simulink library "carnot"  (R2018b)
settings: Solver=VariableStepAuto  StartTime=0.0  StopTime=10.0  RelTol=1e-3
undefined symbols (not defined in the file or in its folder): A, A_earth, acol, Acol, ActPower1, ActPower2, ActPower3, Ad, Ad0, Ar, Au, Au0, Azimuth_Angle, B, Bd, Bd0, Br, Bu, Bu0, C, c1, c2, c3, c33, c4, c5, c6, CarnotCallbacks_Density, CarnotCallbacks_Enthalpy, CarnotCallbacks_Enthalpy2Temperature, CarnotCallbacks_Entropy, CarnotCallbacks_Evaporation_Enthalpy, CarnotCallbacks_GlobalMessageLevel, CarnotCallbacks_Grashof, CarnotCallbacks_Heat_Capacity, CarnotCallbacks_Kinematic_Viscosity, CarnotCallbacks_PMV_PPD, CarnotCallbacks_Prandtl, CarnotCallbacks_Saturation_Property, CarnotCallbacks_Saturation_Temperature, CarnotCallbacks_Saturation_Value_Water, CarnotCallbacks_Specific_Volume, CarnotCallbacks_Thermal_Conductivity, CarnotCallbacks_Vapour_Content, CarnotCallbacks_Vapour_Pressure, Cd, Cdl, Cr, Cu, Davies, Dd, DE_TRY2010_04_averageYear, delta_grd, density, DiameterLastPiece, dl, DPConstant, DPLinear, DPQuadratic, Dr ... (+59)
libraries: $bdroot x429, simulink x36, simulink_extras x12
(part 19 of 22)

== system carnot/Storage/Thermal/Storage_Type_5 ==
  note: Domestic hot water heat exchanger
  note: pipe connection to charge DHW section
  note: pipe connection for house heating
  note: pipe connection to charge house heating section
  note: heat exchanger solar
  note: heat exchanger for DHW circulation
  Tamb : Inport
  THB_dhw : Inport  Port=2
  THB_chg_up : Inport  Port=3
  THB_dis_mid : Inport  Port=4
  THB_chg_mid : Inport  Port=5
  THB_hx_low : Inport  Port=6
  THB_circ : Inport  Port=7
  Pel : Inport  Port=8
  Constant_THB : $bdroot/Source/Simple/Constant_THB  t=20  mdot=0  p=1e5  mID=No Pressure Drop  fluid=Water  mix=0  mix2=0  mix3=0  dia=0.02  hgt=0
  CreateSdat : $bdroot/Basic/Thermal_Models/CreateSdat  volume=volume  stgtype=stgtype
  Electric_Heating_1 : $bdroot/Storage/Thermal/Storage_Ports/Electric_Heating  hin=heater1start  hout=heater1end  nodes=nodes
  HX_EN12977_1 : $bdroot/Storage/Thermal/Storage_Ports/HX_EN12977  h_in=hx1inlet  h_out=hx1outlet  hgt=hgt  dia=hx1dia  height=-0.70492  ua0=hx1uac  uam=hx1uam  uat=hx1uat  uat2=hx1_uat2  dplin=hx1dplin  dpqua=hx1dpqua  nodes=nodes
  HX_EN12977_2 : $bdroot/Storage/Thermal/Storage_Ports/HX_EN12977  h_in=hx2inlet  h_out=hx2outlet  hgt=hgt  dia=hx2dia  height=1.7623  ua0=hx2uac  uam=hx2uam  uat=hx2uat  uat2=hx2_uat2  dplin=hx2dplin  dpqua=hx2dpqua  nodes=nodes
  HX_EN12977_3 : Subsystem  mask(heat exchanger for storage, data EN 12977){h_in=hx3inlet, h_out=hx3outlet, hgt=hgt, dia=hx3dia, height=0.17623, ua0=hx3uac, uam=hx3uam, uat=hx3uat, uat2=hx3_uat2, dplin=hx3dplin, dpqua=hx3dpqua, nodes=nodes}
      mask prompts: h_in "relative height of inlet"; h_out "relative height of outlet"; hgt "Height of storage in m"; dia "Diameter of HX pipe [m]"; height "Height difference inlet-outlet [m]"; ua0 "uac: heat transfer coefficient [W/K /(kg/s) /(°C)]"; uam "uam: massflow dependent heat transfer [-]"; uat "uat: temperature dependent heat transfer [-]"; uat2 "uat2: temperature difference dependent heat transfer [-]"; dplin "Pressure drop coefficient dplin [Pa/(kg/s)]"; dpqua "Pressure drop coefficient dpqua [Pa/(kg/s)²]"; nodes "number of nodes"
      mask help:
      | The block transforms the incoming THV vector to a vector which the storage interprets as a heat exchanger.
      | Give inlet and outlet as a relative position 0=bottom to 1=top
      | The heat transfer is calculated by:
      | UA = uac * mdot^uam *
      |           ((Theatexchanger+Tstorage)/2)^uat *
      |           (Theatexchanger-Tstorage)^uat2
      mask init: same as carnot/Storage/Thermal/Storage_Ports/HX_EN12977
      mask Help: web(['file:///' fullfile(path_carnot('help'),'StoragePorts_HeatExchangerModels.html')],'-helpbrowser')
      mask TypeOptions dia: Pressure_Drop_StorageHX/dia
      mask TypeOptions height: Pressure_Drop_StorageHX/hgt
      mask TypeOptions ua0: sfun_storage_heatexchanger/p1
      mask TypeOptions uam: sfun_storage_heatexchanger/p2
      mask TypeOptions uat: sfun_storage_heatexchanger/p3
      mask TypeOptions uat2: sfun_storage_heatexchanger/p4
      mask TypeOptions dplin: Pressure_Drop_StorageHX/dplin
      mask TypeOptions dpqua: Pressure_Drop_StorageHX/dpqua
      mask TypeOptions nodes: sfun_storage_heatexchanger/nodes
      mask DialogControl ParameterTabVar0 Prompt: Geometry
      mask DialogControl ParameterTabVar01 Prompt: Heat transfer
      mask DialogControl ParameterTabVar012 Prompt: Pressure drop
      mask DialogControl ParameterTabVar0123 Prompt: Calculation
      mask Display: disp('HX EN12977')
  Pipe_Connection_1 : $bdroot/Storage/Thermal/Storage_Ports/Pipe_Connection  h_in=pipe1inlet  h_out=pipe1outlet  hgt=hgt  dpipe=pipe1dia  dstg=dia  height=-0.17623  nodes=nodes
  Pipe_Connection_2 : $bdroot/Storage/Thermal/Storage_Ports/Pipe_Connection  h_in=pipe2inlet  h_out=pipe2outlet  hgt=hgt  dpipe=pipe2dia  dstg=dia  height=0.17623  nodes=nodes
  Pipe_Connection_3 : $bdroot/Storage/Thermal/Storage_Ports/Pipe_Connection  h_in=pipe3inlet  h_out=pipe3outlet  hgt=hgt  dpipe=pipe3dia  dstg=dia  height=-0.70492  nodes=nodes
  T_Sensor_Surface : $bdroot/Control/T_Sensor_Surface  pos=Tsensor  tdel=10  t0=mean(tini)
  select_T : Selector  InputPortWidth=nodes  IndexOptions=Index vector (dialog)  Indices=[1 3 5 7 9 11 13 15 17 19]  OutputSizes=1
  sfun_storageTnodes : $bdroot/Basic/Thermal_Models/sfun_storageTnodes  uloss=uwall  ubot=ubot  utop=utop  cond=axcond  volume=volume  dia=dia  standing=standing cylinder  tini=tini  nodes=nodes  nconnect=7  elimthermocline=2  condinvtc=1e5
  Sdat : Outport
  Tsensors : Outport  Port=2
  THBdhw : Outport  Port=3
  THBchg_up : Outport  Port=4
  THBdis_mid : Outport  Port=5
  THBchg_mid : Outport  Port=6
  THBhx_low : Outport  Port=7
  THBcirc : Outport  Port=8
  wires:
  Electric_Heating_1/1 -> sfun_storageTnodes/8
  Pel/1 -> CreateSdat/20, Electric_Heating_1/1
  HX_EN12977_3/2(THBout) -> CreateSdat/19, THBcirc/1  "THBoutHX3"
  HX_EN12977_3/1(to_storeT) -> sfun_storageTnodes/7
  THB_circ/1 -> CreateSdat/18, HX_EN12977_3/2(THBin)  "THBinHX3"
  T_Sensor_Surface/1 -> Tsensors/1
  HX_EN12977_1/2 -> CreateSdat/15, THBhx_low/1  "THBoutHX1"
  THB_hx_low/1 -> CreateSdat/14, HX_EN12977_1/2  "THBinHX1"
  Pipe_Connection_3/1 -> sfun_storageTnodes/3
  Pipe_Connection_3/2 -> THBchg_up/1, CreateSdat/9  "THBoutPipe3"
  THB_chg_up/1 -> CreateSdat/8, Pipe_Connection_3/2  "THBinPipe3"
  CreateSdat/1 -> Sdat/1
  sfun_storageTnodes/2 -> T_Sensor_Surface/1, select_T/1, HX_EN12977_2/1, Pipe_Connection_3/1, Pipe_Connection_1/1, HX_EN12977_3/1(from_storeT), HX_EN12977_1/1, Pipe_Connection_2/1  "Tnodes"
  select_T/1 -> CreateSdat/3  "Tnodes"
  HX_EN12977_2/1 -> sfun_storageTnodes/2
  HX_EN12977_2/2 -> CreateSdat/17, THBdhw/1  "THBoutHX2"
  THB_dhw/1 -> CreateSdat/16, HX_EN12977_2/2  "THBinHX2"
  Tamb/1 -> sfun_storageTnodes/1, CreateSdat/1  "Tamb"
  THB_dis_mid/1 -> Pipe_Connection_2/2, CreateSdat/6  "THBinPipe2"
  Pipe_Connection_2/1 -> sfun_storageTnodes/4
  Pipe_Connection_2/2 -> THBdis_mid/1, CreateSdat/7  "THBoutPipe2"
  HX_EN12977_1/1 -> sfun_storageTnodes/6
  THB_chg_mid/1 -> CreateSdat/4, Pipe_Connection_1/2, Electric_Heating_1/2  "THBinPipe1"
  Pipe_Connection_1/1 -> sfun_storageTnodes/5
  Pipe_Connection_1/2 -> THBchg_mid/1, CreateSdat/5  "THBoutPipe1"
  sfun_storageTnodes/1 -> CreateSdat/2  "Energy"
  Constant_THB/1 -> CreateSdat/10, CreateSdat/12, CreateSdat/13, CreateSdat/11

== system carnot/Storage/Thermal/detailed_storage_models ==
  heat_exchanger_storage : Subsystem  mask(storage with heat exchanger){v=[0.002 0.0005], loss=0.1, uh=[500 1], uc=[500 1], uw=[300 1], mat=aluminium, m=[3 0.1], t0=20, dph=[200 100 1], dpc=[20 10 0.5], n=1}
      mask prompts: v "volume [exchanger storage] [m³]"; loss "ua losses [W/K]"; uh "heat transfer in exchanger [constant linear_in_massflow] [W/K]"; uc "heat transfer to storage [constant linear_massflow] [W/K]"; uw "heat transfer to wall [constant linear_in_massflow] [W/K]"; mat "material"; m "[mass_in_kg fraction_exchanger]"; t0 "initial temperature [degree centigrade]"; dph "pressure drop exchanger [linear quadratic lin_T] [Pa]"; dpc "pressure drop storage [linear quadratic lin_T] [Pa]"; n "number of nodes"
      mask help: This block is a heat exchanger, taking the fluid volume of the cold and hot side and the thermal capacity of the walls into account.
      mask init:
      | v = max(0.00001, v);
      | n = max(n,1);
      mask Help: web(fullfile(path_carnot('help'),'heat_exchanger_storage.html'),'-helpbrowser')
      mask TypeOptions mat: aluminium | bronze | cast iron | steel | stainless steel | copper | brass | gravel | granite | glass | PU-foam | glass wool
      mask Display: plot(0,-10,110,95,[30,30,35,65,70,70,65,35,30],[90,60,54,54,60,90,95,95,90],[30,66,34,66,34,66,30],[63,63,68,73,76,81,81])

== system carnot/Storage/Thermal/surface_models ==
  Isolated_Cover : Subsystem  mask(isolated cover){u=0.6}
      mask prompts: u "loss coefficient of isolation [W/(m²*K)]"
      mask help: This is a surface-model for ground storages. It describes the absorption of solar radiation and the heat losses by wind.
      mask Help: web(fullfile(path_carnot('help'),'Isolated_Cover.html'),'-helpbrowser')
  Open_Surface : Subsystem  mask(open surface){albedo=0.6}
      mask prompts: albedo "albedo of the surface [0..1]"
      mask help: This is a surface-model for ground storages. It describes the absorption of solar radiation and the heat losses by wind.
      mask init:
      | albedo = min(1, max(0, albedo));
      mask Help: web(fullfile(path_carnot('help'),'Open_Surface.html'),'-helpbrowser')

== system carnot/Basic/Heat_Transfer/alfa_window_in/Shading ==
  WDB : Inport
  control : Inport  Port=2
  Bus Selector : BusSelector  OutputSignals=Zenith_Angle
  Demux : Demux
  Mux : Mux  Inputs=2
  S-Function : S-Function  FunctionName=venetian  Parameters=bli_a, bli_b, bli_c, bli_d, bli_alpha, bli_refl, shad_type, type_glazing, tau_shad  SFunctionDeploymentMode=off  EnableBusSupport=off
  f_dir : Outport
  f_dfu : Outport  Port=2
  f_g : Outport  Port=3
  f_tau : Outport  Port=4
  wires:
  WDB/1 -> Bus Selector/1
  Bus Selector/1 -> Mux/2  "<Zenith_Angle>"
  control/1 -> Mux/1
  Mux/1 -> S-Function/1
  S-Function/1 -> Demux/1
  Demux/1 -> f_dir/1
  Demux/2 -> f_dfu/1
  Demux/3 -> f_g/1
  Demux/4 -> f_tau/1

== system carnot/Basic/Heat_Transfer/alfa_window_in/Subsystem ==
  note: 1. solar radiation into room (behind window glass layers)
      | 2. absorbed solar radiation flowing from inner window surface into zone
  note: TAUALFA 1-2-3-4 layers,standardized to 1.0,(4 mm float glass, no dirt absorption,97% room absorption)
      | The TAUALFA-Lookup-table is calculated with "taualfa.m"
  note: Assumption:
      | 1. gvalue = gvalue(0)
      | 2. gvalue(teta) / gvalue = tau(teta) / tau(0)
  sun_t : Inport
  In2 : Inport  Port=2
  In3 : Inport  Port=3
  In4 : Inport  Port=4
  In5 : Inport  Port=5
  2-D Lookup Table : Lookup_n-D  BreakpointsForDimension1=[0:10:90]  BreakpointsForDimension2=[1:4]  Table=[1.0000 1.0000 1.0000 1.0000; 0.9996 0.9991 0.9987 0.9983; 0.9979 0.9961 0.9945 0.9929; 0.9937 0.9894 0.9861 0.9836; 0.9839 0.9753 0.9704 0.9680; 0.9608 0.9438 0.9365 0.9361; 0.9061 0.8679 0.8484 0.8413; 0.7755 0.6821 0.6182 0.5717; 0.4807 0.3277 0.2324 0.1688; 0 0 0 0]  InternalRulePriority=Speed  RndMeth=Simplest  InputSameDT=on
  Demux2 : Demux  Outputs=2
  Demux3 : Demux  Outputs=3
  Mux2 : Mux  Inputs=2
  Product{1..3,7..8} (5 alike) : Product  SaturateOnIntegerOverflow=on  RndMeth=Zero  InputSameDT=on  OutDataTypeStr=Inherit: Same as first input
  Product11 : Product  Inputs=3  SaturateOnIntegerOverflow=on  RndMeth=Zero  InputSameDT=on  OutDataTypeStr=Inherit: Same as first input
  Sum4 : Sum  Inputs=+-  SaturateOnIntegerOverflow=on  InputSameDT=on  OutDataTypeStr=Inherit: Same as first input
  Sum5 : Sum  SaturateOnIntegerOverflow=on  InputSameDT=on  OutDataTypeStr=Inherit: Same as first input
  const1 : Constant  Value=gvalue
  numlayer : Constant  Value=numlayer
  tau(0) : Gain  Gain=tauzero  SaturateOnIntegerOverflow=on  OutDataTypeStr=Inherit: Same as input  ParamDataTypeStr=Inherit: Same as input
  tau,dfu - angle : Constant  Value=60
  qdot_abs : Outport
  qdot_sol : Outport  Port=2
  wires:
  In5/1 -> Product3/2
  In2/1 -> Product2/2
  Sum4/1 -> qdot_abs/1
  Demux2/2 -> Product8/1  "tau_norm(60)"
  numlayer/1 -> 2-D Lookup Table/2
  Demux2/1 -> Product7/1  "tau_norm(teta)"
  In4/1 -> Product11/3
  Product11/1 -> Sum4/1  "qdot_room"
  Product7/1 -> Sum5/1
  Sum5/1 -> Product11/2, tau(0)/1
  Product3/1 -> Sum4/2, qdot_sol/1
  Product8/1 -> Sum5/2
  Product2/1 -> Product7/2
  tau(0)/1 -> Product3/1
  tau,dfu - angle/1 -> Mux2/2
  Demux3/3 -> Product1/1  "Idfu_t"
  const1/1 -> Product11/1
  Demux3/2 -> Product2/1  "Idir_t"
  Demux3/1 -> Mux2/1  "teta"
  Mux2/1 -> 2-D Lookup Table/1
  In3/1 -> Product1/2
  sun_t/1 -> Demux3/1
  2-D Lookup Table/1 -> Demux2/1
  Product1/1 -> Product8/2

== system carnot/Basic/Hydraulics/Flow_Mixer_basic/Subsystem ==
  clq_bus : Inport
  Bus Selector10 : BusSelector  OutputSignals=MassFlow,DPConstant,DPLinear,DPQuadratic
  Mux : Mux
  clq : Outport
  wires:
  Mux/1 -> clq/1
  clq_bus/1 -> Bus Selector10/1
  Bus Selector10/4 -> Mux/4  "<DPQuadratic>"
  Bus Selector10/3 -> Mux/3  "<DPLinear>"
  Bus Selector10/2 -> Mux/2  "<DPConstant>"
  Bus Selector10/1 -> Mux/1  "<MassFlow>"

== system carnot/Basic/Hydraulics/Flow_Mixer_basic/Subsystem1 ==
  THB : Inport
  Bus Selector1 : BusSelector  OutputSignals=ID,DPConstant,DPLinear,DPQuadratic
  Mux : Mux
  IDclq : Outport
  wires:
  Bus Selector1/4 -> Mux/4  "<DPQuadratic>"
  Bus Selector1/3 -> Mux/3  "<DPLinear>"
  Bus Selector1/2 -> Mux/2  "<DPConstant>"
  Bus Selector1/1 -> Mux/1  "<ID>"
  Mux/1 -> IDclq/1
  THB/1 -> Bus Selector1/1

== system carnot/Basic/Hydraulics/Flow_Mixer_basic/Subsystem2 ==
  THB : Inport
  Bus Selector1 : BusSelector  OutputSignals=ID,DPConstant,DPLinear,DPQuadratic
  Mux : Mux
  IDclq : Outport
  wires:
  THB/1 -> Bus Selector1/1
  Mux/1 -> IDclq/1
  Bus Selector1/1 -> Mux/1  "<ID>"
  Bus Selector1/2 -> Mux/2  "<DPConstant>"
  Bus Selector1/3 -> Mux/3  "<DPLinear>"
  Bus Selector1/4 -> Mux/4  "<DPQuadratic>"

== system carnot/Basic/Hydraulics/Flow_Mixer_basic/average_1 ==
  In1 : Inport
  In2 : Inport  Port=2
  average2 : Gain  Gain=0.5  SaturateOnIntegerOverflow=on  OutDataTypeStr=Inherit: Same as input  ParamDataTypeStr=Inherit: Same as input
  sum2 : Sum  SaturateOnIntegerOverflow=on  InputSameDT=on  OutDataTypeStr=Inherit: Same as first input
  Out1 : Outport
  wires:
  In1/1 -> sum2/1
  average2/1 -> Out1/1
  sum2/1 -> average2/1
  In2/1 -> sum2/2

== system carnot/Basic/Hydraulics/Flow_Mixer_basic/decrease_ID1 ==
  In1 : Inport
  Abs : Abs
  Bias : Bias  Bias=-1
  Dot Product1 : DotProduct  InputSameDT=on  OutDataTypeStr=Inherit: Inherit via internal rule
  Sign : Signum
  Out1 : Outport
  wires:
  Bias/1 -> Dot Product1/2
  Sign/1 -> Dot Product1/1
  Abs/1 -> Bias/1
  Dot Product1/1 -> Out1/1
  In1/1 -> Sign/1, Abs/1

== system carnot/Basic/Hydraulics/Flow_Mixer_basic/decrease_ID2 ==
  In1 : Inport
  Abs : Abs
  Bias : Bias  Bias=-1
  Dot Product1 : DotProduct  InputSameDT=on  OutDataTypeStr=Inherit: Inherit via internal rule
  Sign : Signum
  Out1 : Outport
  wires:
  In1/1 -> Abs/1, Sign/1
  Dot Product1/1 -> Out1/1
  Abs/1 -> Bias/1
  Sign/1 -> Dot Product1/1
  Bias/1 -> Dot Product1/2

== system carnot/Basic/Hydraulics/Mix_T_Mdot/select1 ==
  In1 : Inport
  Bus Selector1 : BusSelector  OutputSignals=Temperature,MassFlow,Pressure,FluidType,FluidMix
  Mux : Mux  Inputs=5
  Out1 : Outport
  wires:
  Mux/1 -> Out1/1
  In1/1 -> Bus Selector1/1
  Bus Selector1/5 -> Mux/5  "<FluidMix>"
  Bus Selector1/4 -> Mux/4  "<FluidType>"
  Bus Selector1/3 -> Mux/3  "<Pressure>"
  Bus Selector1/2 -> Mux/2  "<MassFlow>"
  Bus Selector1/1 -> Mux/1  "<Temperature>"

== system carnot/Basic/Hydraulics/Mix_T_Mdot/select2 ==
  In1 : Inport
  Bus Selector1 : BusSelector  OutputSignals=Temperature,MassFlow,Pressure,FluidType,FluidMix
  Mux : Mux  Inputs=5
  Out1 : Outport
  wires:
  Bus Selector1/1 -> Mux/1  "<Temperature>"
  Bus Selector1/2 -> Mux/2  "<MassFlow>"
  Bus Selector1/3 -> Mux/3  "<Pressure>"
  Bus Selector1/4 -> Mux/4  "<FluidType>"
  Bus Selector1/5 -> Mux/5  "<FluidMix>"
  In1/1 -> Bus Selector1/1
  Mux/1 -> Out1/1

== system carnot/Basic/Pressure_Drop/Pressure_Drop/calculate_dp ==
  THBin : Inport
  c : Inport  Port=2
  l : Inport  Port=3
  q : Inport  Port=4
  Enable : EnablePort
  Bus Selector : BusSelector  OutputSignals=DPConstant
  Bus Selector2 : BusSelector  OutputSignals=DPLinear
  Bus Selector3 : BusSelector  OutputSignals=DPQuadratic
  Bus Selector5 : BusSelector  OutputSignals=MassFlow
  Math Function : Math  Operator=square  SaturateOnIntegerOverflow=on
  Product : Product
  Product1 : Product
  sum : Sum  SaturateOnIntegerOverflow=on  InputSameDT=on  OutDataTypeStr=Inherit: Same as first input
  sum2 : Sum  SaturateOnIntegerOverflow=on  InputSameDT=on  OutDataTypeStr=Inherit: Same as first input
  sum3 : Sum  SaturateOnIntegerOverflow=on  InputSameDT=on  OutDataTypeStr=Inherit: Same as first input
  sum4 : Sum  Inputs=3  SaturateOnIntegerOverflow=on  InputSameDT=on  OutDataTypeStr=Inherit: Same as first input
  dp : Outport
  con : Outport  Port=2
  lin : Outport  Port=3
  qua : Outport  Port=4
  wires:
  sum3/1 -> qua/1
  sum2/1 -> lin/1
  sum/1 -> con/1
  Product/1 -> sum4/2
  Product1/1 -> sum4/1
  Bus Selector2/1 -> sum2/2  "<DPLinear>"
  Bus Selector/1 -> sum/2  "<DPConstant>"
  Bus Selector3/1 -> sum3/2  "<DPQuadratic>"
  Math Function/1 -> Product1/1
  sum4/1 -> dp/1
  Bus Selector5/1 -> Product/1, Math Function/1  "<MassFlow>"
  THBin/1 -> Bus Selector/1, Bus Selector2/1, Bus Selector3/1, Bus Selector5/1
  l/1 -> Product/2, sum2/1
  c/1 -> sum4/3, sum/1
  q/1 -> Product1/2, sum3/1

== system carnot/Basic/Pressure_Drop/Pressure_Drop_PipeTheory/DP_Geometry ==
  Tnodes : Inport
  mdot : Inport  Port=2
  Enable : EnablePort
  Bus Selector4 : BusSelector  OutputSignals=MassFlow,Pressure,FluidType,FluidMix
  S-Function : S-Function  FunctionName=pipe_PressureDrop  Parameters="dia, len,  rough, nbend"  SFunctionDeploymentMode=off  EnableBusSupport=off
  lin : Outport  OutputWhenDisabled=reset  InitialOutput=0
  qua : Outport  Port=2  OutputWhenDisabled=reset  InitialOutput=0
  dp : Outport  Port=3  OutputWhenDisabled=reset  InitialOutput=0
  wires:
  Tnodes/1 -> S-Function/1
  S-Function/1 -> lin/1
  S-Function/2 -> qua/1
  mdot/1 -> Bus Selector4/1
  Bus Selector4/1 -> S-Function/2  "<MassFlow>"
  Bus Selector4/2 -> S-Function/3  "<Pressure>"
  Bus Selector4/3 -> S-Function/4  "<FluidType>"
  Bus Selector4/4 -> S-Function/5  "<FluidMix>"
  S-Function/3 -> dp/1

== system carnot/Basic/Pressure_Drop/Pressure_Drop_changeD/2//pi//d^2//density ==
  note: sudden increase in diameter (A1 < A2)
      |   for a flow from A1 to A2
      |   zeta = (1 - A1/A2)^2 = (1 - (d1/d2)^2)^2
      | sudden decrease in diameter (A1 < A2)
      |   for a flow from A2 to A1
      |   zeta = 0.5 * (1 - A1/A2)^2 = 0.5 * (1 - (d1/d2)^2)^2
      | dp = zeta * density/2 * w^2
      | dp = c + l*mdot + q*mdot^2    Carnot approach (here c = l = 0)
      | with mdot = Vdot*density = w*A*density  -> w = mdot/A/density
      | dp = zeta * density/2 * mdot^2/A^2/density^2
      | dp = zeta/(2*A^2*density) * mdot^2
      | -> q = zeta/(2*A^2*density)
      | diameter increase:
      |   q = (1 - A1/A2)^2/(2*A1^2*density)
      |   q = (1/A1 - 1/A2)^2 / (2*density)
      |   with A = pi/4*d^2
      |   q = 8/density/pi^2 * (1/d1^2 - 1/d2^2)^2
      | diameter decrease:
      |   q = 0.5*(1 - A1/A2)^2/(2*A1^2*density)
      |   q = 0.5*(1/A1 - 1/A2)^2 / (2*density)
      |   with A = pi/4*d^2
      |   q = 4/density/pi^2 * (1/d1^2 - 1/d2^2)^2
  THB : Inport
  Enable : EnablePort
  Abs : Abs
  Add : Sum  Inputs=+-
  Bus Selector3 : BusSelector  OutputSignals=DiameterLastPiece
  Constant : Constant  Value=dia
  Constant1 : Constant  Value=8
  Constant2 : Constant  Value=4
  Density : $bdroot/Basic/Material_Properties/Density  VariantControl=CarlibClassic  INPUTARGUMENTS=THB  DEBUGLEVEL=DEBUGLEVEL  MAXTOTALWARNINGS=inf  MAXCONSECUTIVEWARNINGS=inf  WRITETOFILE=0  FILENAME='errors.txt'
  Gain : Gain  Gain=pi^2
  Math Function1 : Math  Operator=reciprocal  SaturateOnIntegerOverflow=on
  Math Function2 : Math  Operator=square  SaturateOnIntegerOverflow=on
  Math Function4 : Math  Operator=square  SaturateOnIntegerOverflow=on
  Math Function5 : Math  Operator=reciprocal  SaturateOnIntegerOverflow=on
  Math Function6 : Math  Operator=square  SaturateOnIntegerOverflow=on
  Product : Product  Inputs=/**  RndMeth=Zero
  Relational Operator : RelationalOperator  Operator=>  OutDataTypeStr=boolean  RndMeth=Simplest
  Switch : Switch  Criteria=u2 > Threshold
  qua : Outport
  wires:
  Math Function2/1 -> Product/2
  Switch/1 -> Product/3
  Abs/1 -> Math Function2/1
  Add/1 -> Abs/1
  Math Function6/1 -> Add/2
  Math Function4/1 -> Add/1
  Constant2/1 -> Switch/3
  Constant1/1 -> Switch/1
  Relational Operator/1 -> Switch/2
  Constant/1 -> Math Function5/1, Relational Operator/1
  Math Function5/1 -> Math Function6/1
  Math Function1/1 -> Math Function4/1
  Bus Selector3/1 -> Math Function1/1, Relational Operator/2  "<DiameterLastPiece>"
  Density/1 -> Gain/1
  THB/1 -> Bus Selector3/1, Density/1
  Gain/1 -> Product/1
  Product/1 -> qua/1

== system carnot/Basic/Pressure_Drop/Pressure_Drop_staticHeight/Density_x_Gravity ==
  Tnodes : Inport
  THB : Inport  Port=2
  height : Inport  Port=3
  Enable : EnablePort
  Add : Sum
  Add1 : Sum  Inputs=1
  Bus Selector4 : BusSelector  OutputSignals=Pressure,FluidType,FluidMix,GeodeticHeight
  Constant : Constant  Value=9.81
  Density : $bdroot/Basic/Material_Properties/Density  VariantControl=CarlibClassic  INPUTARGUMENTS=state variables (classic)  DEBUGLEVEL=DEBUGLEVEL  MAXTOTALWARNINGS=inf  MAXCONSECUTIVEWARNINGS=inf  WRITETOFILE=0  FILENAME='errors.txt'
  Product : Product  Inputs=/***  RndMeth=Zero
  Width : Width
  pstat : Outport
  GeodeticHeight : Outport  Port=2
  wires:
  Add1/1 -> pstat/1
  Constant/1 -> Product/3
  Product/1 -> Add1/1
  Density/1 -> Product/4
  Width/1 -> Product/1
  Add/1 -> GeodeticHeight/1
  height/1 -> Product/2, Add/2
  Bus Selector4/4 -> Add/1  "<GeodeticHeight>"
  Tnodes/1 -> Width/1, Density/1
  THB/1 -> Bus Selector4/1
  Bus Selector4/3 -> Density/4  "<FluidMix>"
  Bus Selector4/2 -> Density/3  "<FluidType>"
  Bus Selector4/1 -> Density/2  "<Pressure>"

== system carnot/Basic/Thermal_Models/Combustion_Calculation/exhaust gas ==
  note: gas = 1
      | liquid = 2
      | solid = 3
  ID : Inport
  h : Inport  Port=2
  c : Inport  Port=3
  o : Inport  Port=4
  s : Inport  Port=5
  n : Inport  Port=6
  w : Inport  Port=7
  Demux : Demux
  Multiport Switch : MultiPortSwitch  SaturateOnIntegerOverflow=on  InputSameDT=on
  Terminator : Terminator
  fluid/solid : Subsystem
  gas : Subsystem
  CO2 : Outport
  H2O : Outport  Port=2
  SO2 : Outport  Port=3
  N2 : Outport  Port=4
  wires:
  ID/1 -> Multiport Switch/1
  fluid/solid/1(Out1) -> Multiport Switch/4, Multiport Switch/3
  Multiport Switch/1 -> Demux/1
  Demux/4 -> N2/1
  Demux/3 -> SO2/1
  Demux/2 -> H2O/1
  Demux/1 -> CO2/1
  s/1 -> gas/3(s), fluid/solid/3(s)
  n/1 -> gas/4(n), fluid/solid/4(n)
  h/1 -> gas/2(h), fluid/solid/2(h)
  c/1 -> gas/1(c), fluid/solid/1(c)
  o/1 -> Terminator/1
  w/1 -> fluid/solid/5(w)
  gas/1(Out1) -> Multiport Switch/2

== system carnot/Basic/Thermal_Models/HeatPump_basic/P_el calculus ==
  note: Pel = K4*Tcold_in + K5*Thot_out + K6
  Thot_out : Inport
  Tcold_in : Inport  Port=2
  Add : Sum  Inputs=+++
  Thot_dependancy : Gain  Gain=K(5)  SaturateOnIntegerOverflow=on  OutDataTypeStr=Inherit: Same as input  ParamDataTypeStr=Inherit: Same as input
  Tsource dependancy : Gain  Gain=K(4)  SaturateOnIntegerOverflow=on  OutDataTypeStr=Inherit: Same as input  ParamDataTypeStr=Inherit: Same as input
  constant power : Constant  Value=K(6)
  P_el : Outport
  wires:
  Thot_dependancy/1 -> Add/1
  Thot_out/1 -> Thot_dependancy/1
  Tsource dependancy/1 -> Add/2
  Add/1 -> P_el/1
  Tcold_in/1 -> Tsource dependancy/1
  constant power/1 -> Add/3

== system carnot/Basic/Thermal_Models/HeatPump_basic/model cold side ==
  note: Qdot_h = K1*Tcold_in + K2*Thot_out + K3
      |
      | Qdot_c = -K7*Tcold_in - K8*Thot_out - K9
      |
      | cap_h*dTh/dt = Qdot_h + mdot_h*cp_h*(Th_in-Th) + UA*(Tamb-Th)
      |
      | cap_c*dTc/dt = Qdot_c + mdot_c*cp_c*(Tc_in-Tc) + UA*(Tamb-Tc)
      |
      | cap_h = mass_hot_side * heat_capactiy_hot_side
      |
      | cap_c = mass_cold_side * heat_capactiy_cold_side
  Tcold : Inport
  mdot_cold : Inport  Port=2
  p_cold : Inport  Port=3
  fluid_cold : Inport  Port=4
  mix_cold : Inport  Port=5
  Thot : Inport  Port=6
  Tamb : Inport  Port=7
  command : Inport  Port=8
  1/(m*cp) : Gain  Gain=1/capc
  Add2 : Sum  Inputs=+-
  Add4 : Sum  Inputs=+-
  Heat_Capacity : $bdroot/Basic/Material_Properties/Heat_Capacity  VariantControl=CarlibClassic  INPUTARGUMENTS=state variables (classic)  DEBUGLEVEL=DEBUGLEVEL  MAXTOTALWARNINGS=inf  MAXCONSECUTIVEWARNINGS=inf  WRITETOFILE=0  FILENAME='errors.txt'
  Integrator : Integrator  InitialConditionSource=external  InitialCondition=25
  Product{2..5} (4 alike) : DotProduct  InputSameDT=on  OutDataTypeStr=Inherit: Inherit via internal rule
  Sum1 : Sum  Inputs=---  SaturateOnIntegerOverflow=on  InputSameDT=on  OutDataTypeStr=Inherit: Same as first input
  Sum2 : Sum  Inputs=3  SaturateOnIntegerOverflow=on  InputSameDT=on  OutDataTypeStr=Inherit: Same as first input
  Thot_dependancy : Gain  Gain=K(8)  SaturateOnIntegerOverflow=on  OutDataTypeStr=Inherit: Same as input  ParamDataTypeStr=Inherit: Same as input
  Tsource dependancy : Gain  Gain=K(7)  SaturateOnIntegerOverflow=on  OutDataTypeStr=Inherit: Same as input  ParamDataTypeStr=Inherit: Same as input
  add constant : Subsystem  mask(add constant){c=+1}
      mask prompts: c "constant c"
      mask help: This block adds a constant c to each element of the input vector.
      mask Help: eval('htmlhelp (''chap_4_2a.htm#add_constant'')')
      mask Display: disp('+c');
  const Power1 : Gain  Gain=-1  SaturateOnIntegerOverflow=on  OutDataTypeStr=Inherit: Same as input  ParamDataTypeStr=Inherit: Same as input
  constant power : Constant  Value=K(9)
  losses : Gain  Gain=UA
  Tcold_out : Outport
  mdot*cp : Outport  Port=2
  wires:
  1/(m*cp)/1 -> Integrator/1
  fluid_cold/1 -> Heat_Capacity/3
  mix_cold/1 -> Heat_Capacity/4
  p_cold/1 -> Heat_Capacity/2
  Thot/1 -> Thot_dependancy/1
  Product2/1 -> Product5/1, mdot*cp/1
  Heat_Capacity/1 -> Product2/2
  mdot_cold/1 -> Product2/1
  Add2/1 -> losses/1
  Tcold/1 -> Add4/1, Heat_Capacity/1, Tsource dependancy/1
  Tsource dependancy/1 -> Sum1/1
  Thot_dependancy/1 -> Sum1/2
  constant power/1 -> Sum1/3
  Sum1/1 -> Product4/2  "Qdot_hot"
  Tamb/1 -> Add2/1, Integrator/2
  command/1 -> Product4/1, const Power1/1
  losses/1 -> Product3/2
  add constant/1(Out1) -> Product3/1
  const Power1/1 -> add constant/1(In1)
  Add4/1 -> Product5/2
  Sum2/1 -> 1/(m*cp)/1
  Product3/1 -> Sum2/3
  Product4/1 -> Sum2/2
  Product5/1 -> Sum2/1
  Integrator/1 -> Tcold_out/1, Add2/2, Add4/2

== system carnot/Basic/Thermal_Models/HeatPump_basic/model hot side ==
  note: Qdot_h = K1*Tcold_in + K2*Thot_out + K3
      |
      | Qdot_c = -K7*Tcold_in - K8*Thot_out - K9
      |
      | cap_h*dTh/dt = Qdot_h + mdot_h*cp_h*(Th_in-Th) + UA*(Tamb-Th)
      |
      | cap_c*dTc/dt = Qdot_c + mdot_c*cp_c*(Tc_in-Tc) + UA*(Tamb-Tc)
      |
      | cap_h = mass_hot_side * heat_capactiy_hot_side
      |
      | cap_c = mass_cold_side * heat_capactiy_cold_side
  Tcold : Inport
  Thot : Inport  Port=2
  mdot_hot : Inport  Port=3
  p_hot : Inport  Port=4
  fluid_hot : Inport  Port=5
  mix_hot : Inport  Port=6
  Tamb : Inport  Port=7
  command : Inport  Port=8
  1/(m*cp) : Gain  Gain=1/caph
  Add2 : Sum  Inputs=+-
  Add4 : Sum  Inputs=+-
  Bias : Bias  Bias=1
  Heat_Capacity : $bdroot/Basic/Material_Properties/Heat_Capacity  VariantControl=CarlibClassic  INPUTARGUMENTS=state variables (classic)  DEBUGLEVEL=DEBUGLEVEL  MAXTOTALWARNINGS=inf  MAXCONSECUTIVEWARNINGS=inf  WRITETOFILE=0  FILENAME='errors.txt'
  Integrator : Integrator  InitialConditionSource=external  InitialCondition=25
  Product{2..5} (4 alike) : DotProduct  InputSameDT=on  OutDataTypeStr=Inherit: Inherit via internal rule
  Sum1 : Sum  Inputs=+++  SaturateOnIntegerOverflow=on  InputSameDT=on  OutDataTypeStr=Inherit: Same as first input
  Sum2 : Sum  Inputs=+++  SaturateOnIntegerOverflow=on  InputSameDT=on  OutDataTypeStr=Inherit: Same as first input
  Thot_dependancy : Gain  Gain=K(2)  SaturateOnIntegerOverflow=on  OutDataTypeStr=Inherit: Same as input  ParamDataTypeStr=Inherit: Same as input
  Tsource dependancy : Gain  Gain=K(1)  SaturateOnIntegerOverflow=on  OutDataTypeStr=Inherit: Same as input  ParamDataTypeStr=Inherit: Same as input
  const Power1 : Gain  Gain=-1  SaturateOnIntegerOverflow=on  OutDataTypeStr=Inherit: Same as input  ParamDataTypeStr=Inherit: Same as input
  constant power : Constant  Value=K(3)
  losses : Gain  Gain=UA
  mdot*cp : Outport
  Thot_out : Outport  Port=2
  wires:
  Integrator/1 -> Add2/2, Thot_dependancy/1, Add4/2, Thot_out/1
  Product5/1 -> Sum2/1
  Product4/1 -> Sum2/2
  Product3/1 -> Sum2/3
  1/(m*cp)/1 -> Integrator/1
  Sum2/1 -> 1/(m*cp)/1
  Add4/1 -> Product5/2
  const Power1/1 -> Bias/1
  Bias/1 -> Product3/1
  losses/1 -> Product3/2
  command/1 -> const Power1/1, Product4/1
  Tamb/1 -> Integrator/2, Add2/1
  Sum1/1 -> Product4/2  "Qdot_hot"
  constant power/1 -> Sum1/3
  Thot_dependancy/1 -> Sum1/2
  Tsource dependancy/1 -> Sum1/1
  Tcold/1 -> Tsource dependancy/1
  Add2/1 -> losses/1
  mdot_hot/1 -> Product2/1
  Heat_Capacity/1 -> Product2/2
  Product2/1 -> Product5/1, mdot*cp/1
  Thot/1 -> Add4/1, Heat_Capacity/1
  p_hot/1 -> Heat_Capacity/2
  mix_hot/1 -> Heat_Capacity/4
  fluid_hot/1 -> Heat_Capacity/3

== system carnot/Basic/Thermal_Models/House_OneNodeModel/Troom_calc ==
  Qdot : Inport
  A : Constant  Value=A
  Product : Product  Inputs=*//
  Switch : Switch  Criteria=u2 > Threshold
  Tini : Constant  Value=tini
  Transfer Fcn : TransferFcn  Commented=on  Denominator=[1 1]
  add_Tini : Bias  Bias=tini
  capa : Constant  Value=capa
  dtroom : Constant  Value=dtroom
  energy : Integrator  LimitOutput=on  UpperSaturationLimit=dtroom  LowerSaturationLimit=min(-dtroom, -0.01)
  sum : Sum  Inputs=1  SaturateOnIntegerOverflow=on  InputSameDT=on  OutDataTypeStr=Inherit: Same as first input
  Troom : Outport
  wires:
  add_Tini/1 -> Switch/1
  dtroom/1 -> Switch/2
  Tini/1 -> Switch/3
  capa/1 -> Product/3
  A/1 -> Product/2
  Qdot/1 -> sum/1
  Switch/1 -> Troom/1  "Troom"
  energy/1 -> add_Tini/1
  Product/1 -> energy/1
  sum/1 -> Product/1

== system carnot/Basic/Thermal_Models/Room_Node/Sensitive room temperature ==
  note: Sensitive temperature
  Tr : Inport
  Tc : Inport  Port=2
  1-share_c : Gain  Gain=1-share_c  SaturateOnIntegerOverflow=on  OutDataTypeStr=Inherit: Same as input  ParamDataTypeStr=Inherit: Same as input
  Sum : Sum  SaturateOnIntegerOverflow=on  InputSameDT=on  OutDataTypeStr=Inherit: Same as first input
  share_c : Gain  Gain=share_c  SaturateOnIntegerOverflow=on  OutDataTypeStr=Inherit: Same as input  ParamDataTypeStr=Inherit: Same as input
  Ts : Outport
  wires:
  Tr/1 -> 1-share_c/1
  Tc/1 -> share_c/1
  share_c/1 -> Sum/1  "Tc"
  1-share_c/1 -> Sum/2  "Tr"
  Sum/1 -> Ts/1

== system carnot/Basic/Thermal_Models/Room_Node/convective_node ==
  note: (m^3/s)
  note: (kg/s)
  note: (W)
  note: (°C)
  note: (kg water / kg air)
  note: (kg/s)
  note: (kg/s)
  note: (m^3/s)
  note: (1/s)
  note: CONVECTIVE node: absolute air mass, humidity mass, CO2 mass and air temperature in a zone
  note: (kg/m^3)
  note: SIMPLIFICATIONS:
      | 1) air in zone is incompressible
      | 2) density and heat-capacity are constant
  note: (J/(kg*K))
  note: (kg CO2 / kg air)
  note: (N/m^2)
  Qdotc : Inport
  D_mdot_air : Inport  Port=2
  D_mdot_H2O : Inport  Port=3
  D_mdot_CO2 : Inport  Port=4
  Vdot_out2in : Inport  Port=5
  Vdot_in2out : Inport  Port=6
  (1/m^3)1 : Constant  Value=heatperfect
  (m^3) : Constant  Value=zoneairvolume
  Constant : Constant  Value=AirPressure
  Constant1 : Constant  Value=calc_p  mask{calc_p=off}
      mask prompts: calc_p "Calculate Pressure"
  Multiport Switch : MultiPortSwitch  Inputs=2  SaturateOnIntegerOverflow=on  InputSameDT=on
  PressureCalculation : Subsystem
  Repeating Sequence : simulink/Sources/Repeating Sequence  rep_seq_t=lookuptime  rep_seq_y=lookupvalue
  Sum : Sum  SaturateOnIntegerOverflow=on  InputSameDT=on  OutDataTypeStr=Inherit: Same as first input
  Switch : Switch  Criteria=u2 > Threshold  Threshold=0.5
  Tair : Integrator  InitialCondition=zonestartTEMP
  density_air : Constant  Value=density(zonestartTEMP, AirPressure, 2, rel_hum2x(zonestartTEMP, AirPressure,zonestartWATER))
  gain : Gain  Gain=0.5  SaturateOnIntegerOverflow=on  OutDataTypeStr=Inherit: Same as input  ParamDataTypeStr=Inherit: Same as input
  heat_capacity_air : Constant  Value=heat_capacity(zonestartTEMP, AirPressure, 2, rel_hum2x(zonestartTEMP, AirPressure,zonestartWATER))
  m_CO2 : Integrator  InitialCondition="CO2norm*1.529*zoneairvolume   % kg CO2 in zone volume"  LimitOutput=on  LowerSaturationLimit=0
  m_H2O : Integrator  InitialCondition="rel_hum2x(zonestartTEMP, 1e5, zonestartWATER)*1.18*zoneairvolume    % kg H2O in zone volume"  LimitOutput=on  LowerSaturationLimit=0
  x1 : Product  Inputs=*//  SaturateOnIntegerOverflow=on  InputSameDT=on  OutDataTypeStr=Inherit: Same as first input
  x2 : Product  Inputs=**/  SaturateOnIntegerOverflow=on  InputSameDT=on  OutDataTypeStr=Inherit: Same as first input
  x3 : Product  Inputs=*///  SaturateOnIntegerOverflow=on  InputSameDT=on  OutDataTypeStr=Inherit: Same as first input
  x4 : Product  Inputs=/*  SaturateOnIntegerOverflow=on  InputSameDT=on  OutDataTypeStr=Inherit: Same as first input
  Tc : Outport
  x_H2O : Outport  Port=2
  x_CO2 : Outport  Port=3
  rho : Outport  Port=4
  cp : Outport  Port=5
  p : Outport  Port=6
  nair_out : Outport  Port=7
  wires:
  Constant/1 -> Switch/3
  Switch/1 -> p/1
  PressureCalculation/1(p) -> Switch/1
  Constant1/1 -> Switch/2, PressureCalculation/Enable
  D_mdot_air/1 -> PressureCalculation/1(D_mdot_air)
  Sum/1 -> gain/1
  density_air/1 -> x3/3, rho/1, x2/3, x1/3, PressureCalculation/2(density)
  Qdotc/1 -> x3/1
  gain/1 -> x4/2
  Vdot_out2in/1 -> Sum/1
  Vdot_in2out/1 -> Sum/2
  x4/1 -> nair_out/1
  m_H2O/1 -> x1/1
  D_mdot_CO2/1 -> m_CO2/1
  D_mdot_H2O/1 -> m_H2O/1
  x1/1 -> x_H2O/1
  heat_capacity_air/1 -> x3/4, cp/1
  m_CO2/1 -> x2/1
  x3/1 -> Tair/1
  Tair/1 -> Multiport Switch/2
  x2/1 -> x_CO2/1
  Multiport Switch/1 -> Tc/1, PressureCalculation/4(T)
  (1/m^3)1/1 -> Multiport Switch/1
  Repeating Sequence/1 -> Multiport Switch/3
  (m^3)/1 -> x3/2, x4/1, x2/2, x1/2, PressureCalculation/3(zoneairvolume)

== system carnot/Basic/Thermal_Models/Room_Node/radiative_node ==
  note: RADIATIVE node
  Qdotr : Inport
  (1/m^3)1 : Constant  Value=heatperfect
  Gain : Gain  Gain=1/timeconst
  Integrator : Integrator  InitialCondition=zonestartTEMP
  Multiport Switch : MultiPortSwitch  Inputs=2  SaturateOnIntegerOverflow=on  InputSameDT=on
  Repeating Sequence : simulink/Sources/Repeating Sequence  rep_seq_t=lookuptime  rep_seq_y=lookupvalue
  Tr : Outport
  wires:
  Multiport Switch/1 -> Tr/1
  Integrator/1 -> Multiport Switch/2
  (1/m^3)1/1 -> Multiport Switch/1
  Qdotr/1 -> Gain/1
  Gain/1 -> Integrator/1
  Repeating Sequence/1 -> Multiport Switch/3

== system carnot/Basic/Thermal_Models/Window/lambda_window ==
  note: Timeconstant of window is calculated
      | in the mask initialization
  note: Heat conduction in a window (ONLY SURFACE LAYER CONNECTABLE)
  qdots1 : Inport
  qdots2 : Inport  Port=2
  Gain : Gain  Gain=Rwin
  Gain1 : Gain  Gain=Rwin
  Sum1 : Sum  SaturateOnIntegerOverflow=on  InputSameDT=on  OutDataTypeStr=Inherit: Same as first input
  Sum3 : Sum  SaturateOnIntegerOverflow=on  InputSameDT=on  OutDataTypeStr=Inherit: Same as first input
  Transfer Fcn (with initial outputs)1 : simulink_extras/Additional Linear/Transfer Fcn (with initial outputs)  N=[1]  D=[timeconst 1]  Y0=t0  U0=t0
  Transfer Fcn (with initial outputs)2 : simulink_extras/Additional Linear/Transfer Fcn (with initial outputs)  N=[1]  D=[timeconst 1]  Y0=t0  U0=t0
  Ts1 : Outport
  Ts2 : Outport  Port=2
  wires:
  Gain1/1 -> Sum1/2
  Gain/1 -> Sum3/1
  Sum1/1 -> Transfer Fcn (with initial outputs)2/1
  qdots2/1 -> Gain1/1
  Sum3/1 -> Transfer Fcn (with initial outputs)1/1
  qdots1/1 -> Gain/1
  Transfer Fcn (with initial outputs)1/1 -> Ts1/1, Sum1/1
  Transfer Fcn (with initial outputs)2/1 -> Sum3/2, Ts2/1

== system carnot/Hydraulics/Valve/relFlowCoefficientFunction/EqualPercentageCharacteristic ==
  note: Equal percentage characteristics of the valve:
      | psi = psi_0 * e^(n*h)
      | with
      | n = ln(1/psi_0) inclination of the characteristics
      | the relative flow coefficient is:
      | psi = psi_0 * (1/psi_0)^h)
  h : Inport
  Action Port : ActionPort
  Math Function : Math  Operator=pow  SaturateOnIntegerOverflow=on
  Product : Product  Inputs=*/
  Product1 : Product
  const : Constant
  psi_0 : Constant  Value=psi_0
  psi : Outport
  wires:
  Math Function/1 -> Product1/1
  h/1 -> Math Function/2
  Product/1 -> Math Function/1
  psi_0/1 -> Product/2, Product1/2
  const/1 -> Product/1
  Product1/1 -> psi/1  "psi"

== system carnot/Hydraulics/Valve/relFlowCoefficientFunction/LinearCharacteristic ==
  note: Linear characteristics of the valve:
      | psi = psi_0 + (1-psi_0)*h
      | with
      | h = H/H100 relative opening
      | psi_0 relative flow coeff. at h = 0
  h : Inport
  Action Port : ActionPort
  Add : Sum  Inputs=+-
  Add1 : Sum  Inputs=2
  Product : Product
  const : Constant
  psi_0 : Constant  Value=psi_0
  psi : Outport
  wires:
  Add1/1 -> psi/1  "psi"
  Product/1 -> Add1/1
  h/1 -> Product/1
  Add/1 -> Product/2
  psi_0/1 -> Add/2, Add1/2
  const/1 -> Add/1

== system carnot/Hydraulics/Valve/relFlowCoefficientFunction/defaultLinear ==
  note: Linear characteristics of the valve:
      | psi = psi_0 + (1-psi_0)*h
      | with
      | h = H/H100 relative opening
      | psi_0 relative flow coeff. at h = 0
  h : Inport
  Action Port : ActionPort
  Add : Sum  Inputs=+-
  Add1 : Sum  Inputs=2
  Product : Product
  const : Constant
  psi_0 : Constant  Value=psi_0
  psi : Outport
  wires:
  const/1 -> Add/1
  psi_0/1 -> Add1/2, Add/2
  Add/1 -> Product/2
  h/1 -> Product/1
  Product/1 -> Add1/1
  Add1/1 -> psi/1  "psi"

== system carnot/Load/Houses/House_simple/AirComposition ==
  THBvent : Inport
  RDB : Inport  Port=2
  Enable : EnablePort
  Bus Creator : BusCreator  Inputs=3
  Bus Selector : BusSelector  OutputSignals=Massflow_CO2,Massflow_H2O,Massflow_VOC
  Terminator : Terminator
  TransferFcn CO2 : simulink_extras/Additional Linear/Transfer Fcn (with initial states)  N=[1]  D="[1  1]"  X0=.5
  TransferFcn H2O : simulink_extras/Additional Linear/Transfer Fcn (with initial states)  N=[1]  D="[1  1]"  X0=.5
  TransferFcn VOC : simulink_extras/Additional Linear/Transfer Fcn (with initial states)  N=[1]  D="[1  1]"  X0=.5
  AirComp : Outport
  wires:
  THBvent/1 -> Terminator/1
  TransferFcn VOC/1 -> Bus Creator/3
  TransferFcn H2O/1 -> Bus Creator/2
  TransferFcn CO2/1 -> Bus Creator/1
  Bus Creator/1 -> AirComp/1
  Bus Selector/2 -> TransferFcn H2O/1  "<Massflow_H2O>"
  Bus Selector/3 -> TransferFcn VOC/1  "<Massflow_VOC>"
  Bus Selector/1 -> TransferFcn CO2/1  "<Massflow_CO2>"
  RDB/1 -> Bus Selector/1

== system carnot/Source/Boiler/Condensing_Boiler/SelectTefficiency ==
  Tout : Inport
  Tin : Inport  Port=2
  Constant : Constant  Value=whichTforEfficiency
  Gain1 : Gain  Gain=1/2
  Multiport Switch : MultiPortSwitch
  Sum : Sum
  Tmean : Outport
  Teff : Outport  Port=2
  wires:
  Tin/1 -> Multiport Switch/3, Sum/1
  Tout/1 -> Sum/2, Multiport Switch/4
  Sum/1 -> Gain1/1
  Multiport Switch/1 -> Teff/1
  Gain1/1 -> Multiport Switch/2, Tmean/1  "Tmean"
  Constant/1 -> Multiport Switch/1

== system carnot/Source/Boiler/Condensing_Boiler/limitCtrl ==
  In1 : Inport
  Constant : Constant  Value=0
  Saturation : Saturate  UpperLimit=1  LowerLimit=0
  Switch : Switch  Threshold=relQdotMin
  Out1 : Outport
  wires:
  In1/1 -> Switch/2, Switch/1
  Switch/1 -> Saturation/1
  Constant/1 -> Switch/3
  Saturation/1 -> Out1/1

== system carnot/Source/Chiller/Absorption_Chiller_LookUp/Lookup_table Q_hot + Q_cold + Recooling ==
  T_GEN_IN : Inport
  T_RC_IN : Inport  Port=2
  T_COLD_IN : Inport  Port=3
  control : Inport  Port=4
  Divide : Product  Inputs=/**
  HT_cap : simulink_extras/Additional Linear/Transfer Fcn (with initial states)  N=[1]  D="[21.55  1]"  X0=0
  NTDeadTime : Subsystem
  Product : Product  RndMeth=Zero
  Product1 : Product  Inputs=3  RndMeth=Zero
  Product2 : Product  RndMeth=Zero
  Q_cold_cap : simulink_extras/Additional Linear/Transfer Fcn (with initial states)  N=[1]  D="[52.356  1]"  X0=0
  Saturation : Saturate  UpperLimit=inf  LowerLimit=0
  Saturation1 : Saturate  UpperLimit=inf  LowerLimit=0
  Saturation2 : Saturate  UpperLimit=inf  LowerLimit=0
  Saturation3 : Saturate  UpperLimit=inf  LowerLimit=eps(10)  ZeroCross=off
  lookup_table_Q_cold : Lookup_n-D  NumberOfTableDimensions=3  BreakpointsForDimension1=data.cooling_T_heating  BreakpointsForDimension2=data.cooling_T_recooling  BreakpointsForDimension3=data.cooling_T_cooling  BreakpointsForDimension4=[1:2]  Table=data.cooling_Qdot  InputSameDT=on
  lookup_table_Q_hot : Lookup_n-D  NumberOfTableDimensions=3  BreakpointsForDimension1=data.heating_T_heating  BreakpointsForDimension2=data.heating_T_recooling  BreakpointsForDimension3=data.heating_T_cooling  BreakpointsForDimension4=[1:2]  Table=data.heating_Qdot  InputSameDT=on
  lookup_table_Q_recooling : Lookup_n-D  NumberOfTableDimensions=3  BreakpointsForDimension1=data.recooling_T_heating  BreakpointsForDimension2=data.recooling_T_recooling  BreakpointsForDimension3=data.recooling_T_cooling  BreakpointsForDimension4=[1:2]  Table=data.recooling_Qdot  InputSameDT=on
  recooling_cap : simulink_extras/Additional Linear/Transfer Fcn (with initial states)  N=[1]  D="[104.17  1]"  X0=0
  runtime_AC : Subsystem  TreatAsAtomicUnit=on
      mask help: This block counts the time if input is set to one, it stops counting if input is zero and continues when input rises to one again.
      mask Help: eval('filetest (''manual.htm#count_working_time'')')
  Q_hot_kW : Outport
  Q_cold_kW : Outport  Port=2
  Q_recooling_kW : Outport  Port=3
  COP : Outport  Port=4
  wires:
  T_COLD_IN/1 -> lookup_table_Q_cold/3, lookup_table_Q_recooling/3, lookup_table_Q_hot/3
  T_RC_IN/1 -> lookup_table_Q_cold/2, lookup_table_Q_recooling/2, lookup_table_Q_hot/2
  T_GEN_IN/1 -> lookup_table_Q_cold/1, lookup_table_Q_recooling/1, NTDeadTime/2(T_HT_IN), lookup_table_Q_hot/1
  lookup_table_Q_hot/1 -> Saturation/1
  control/1 -> Product/2, Product1/1, runtime_AC/1(control_AC), Product2/1
  runtime_AC/1(runtime) -> NTDeadTime/1(control_AC_runtime)
  Product/1 -> HT_cap/1
  Product1/1 -> Q_cold_cap/1
  HT_cap/1 -> Q_hot_kW/1, Saturation3/1
  Q_cold_cap/1 -> Q_cold_kW/1, Divide/3
  lookup_table_Q_cold/1 -> Saturation1/1
  recooling_cap/1 -> Q_recooling_kW/1
  Product2/1 -> recooling_cap/1
  lookup_table_Q_recooling/1 -> Saturation2/1
  Saturation/1 -> Product/1
  Saturation1/1 -> Product1/3
  Saturation2/1 -> Product2/2
  Divide/1 -> COP/1
  NTDeadTime/1(Q_cold_on) -> Divide/2, Product1/2
  Saturation3/1 -> Divide/1

== system carnot/Source/Chiller/Absorption_Chiller_LookUp/cooling ==
  Q_cold : Inport
  THB_COLD_IN : Inport  Port=2  OutDataTypeStr=Bus: THB
  Bus Assignment : BusAssignment  AssignedSignals=Temperature
  Bus Selector : BusSelector  OutputSignals=Temperature,Pressure,FluidType,FluidMix,MassFlow
  Heat_Capacity : $bdroot/Basic/Material_Properties/Heat_Capacity  VariantControl=CarlibClassic  INPUTARGUMENTS=state variables (classic)  DEBUGLEVEL=DEBUGLEVEL  MAXTOTALWARNINGS=inf  MAXCONSECUTIVEWARNINGS=inf  WRITETOFILE=0  FILENAME='errors.txt'
  Pipe : $bdroot/Hydraulics/Pipe  dia=0.02  len=10  hgt=5  uloss=100/20/10  cond=0  cwall=1000  t0=20  lin=100/0.2  qua=100/0.2^2  nodes=10
  Product : Product  Inputs=//*  SaturateOnIntegerOverflow=on  RndMeth=Zero  InputSameDT=on  OutDataTypeStr=Inherit: Same as first input
  Sum2 : Sum  Inputs=+-  InputSameDT=on  OutDataTypeStr=Inherit: Same as first input
  const1 : Constant  Value=20
  isinf : MATLAB Function  TreatAsAtomicUnit=on
  isnan : MATLAB Function  TreatAsAtomicUnit=on
  THB_COLD_OUT : Outport
  wires:
  Heat_Capacity/1 -> Product/1
  THB_COLD_IN/1 -> Bus Assignment/1, Bus Selector/1
  Bus Selector/1 -> Sum2/1, Heat_Capacity/1  "<Temperature>"
  Bus Selector/2 -> Heat_Capacity/2  "<Pressure>"
  Bus Selector/3 -> Heat_Capacity/3  "<FluidType>"
  Bus Selector/4 -> Heat_Capacity/4  "<FluidMix>"
  isnan/1(y) -> isinf/1(u)
  Product/1 -> isnan/1(u)
  isinf/1(y) -> Sum2/2
  Bus Selector/5 -> Product/2  "<MassFlow>"
  Sum2/1 -> Bus Assignment/2
  Pipe/1 -> THB_COLD_OUT/1
  Bus Assignment/1 -> Pipe/2
  const1/1 -> Pipe/1
  Q_cold/1 -> Product/3

== system carnot/Source/Chiller/Absorption_Chiller_LookUp/generator ==
  THB_GEN_IN : Inport
  Q_hot : Inport  Port=2
  Bus Assignment : BusAssignment  AssignedSignals=Temperature
  Bus Selector : BusSelector  OutputSignals=Temperature,Pressure,FluidType,FluidMix,MassFlow
  Constant2 : Constant  Value=20
  Heat_Capacity : $bdroot/Basic/Material_Properties/Heat_Capacity  VariantControl=CarlibClassic  INPUTARGUMENTS=state variables (classic)  DEBUGLEVEL=DEBUGLEVEL  MAXTOTALWARNINGS=inf  MAXCONSECUTIVEWARNINGS=inf  WRITETOFILE=0  FILENAME='errors.txt'
  Pipe : $bdroot/Hydraulics/Pipe  dia=0.02  len=10  hgt=5  uloss=100/20/10  cond=0  cwall=1000  t0=20  lin=100/0.2  qua=100/0.2^2  nodes=10
  Product3 : Product  Inputs=//*  SaturateOnIntegerOverflow=on  RndMeth=Zero  InputSameDT=on  OutDataTypeStr=Inherit: Same as first input
  Sum2 : Sum  Inputs=+-  InputSameDT=on  OutDataTypeStr=Inherit: Same as first input
  isinf : MATLAB Function  TreatAsAtomicUnit=on
  isnan : MATLAB Function  TreatAsAtomicUnit=on
  THV_GEN_OUT : Outport
  wires:
  Product3/1 -> isnan/1(u)
  Heat_Capacity/1 -> Product3/1
  Bus Selector/1 -> Sum2/1, Heat_Capacity/1  "<Temperature>"
  Q_hot/1 -> Product3/3
  isnan/1(y) -> isinf/1(u)
  isinf/1(y) -> Sum2/2
  Sum2/1 -> Bus Assignment/2
  Pipe/1 -> THV_GEN_OUT/1
  Constant2/1 -> Pipe/1
  THB_GEN_IN/1 -> Bus Assignment/1, Bus Selector/1
  Bus Selector/2 -> Heat_Capacity/2  "<Pressure>"
  Bus Selector/3 -> Heat_Capacity/3  "<FluidType>"
  Bus Selector/4 -> Heat_Capacity/4  "<FluidMix>"
  Bus Selector/5 -> Product3/2  "<MassFlow>"
  Bus Assignment/1 -> Pipe/2

== system carnot/Source/Chiller/Absorption_Chiller_LookUp/recooling ==
  Q_recooling : Inport
  THB_RC_IN : Inport  Port=2
  Bus Assignment : BusAssignment  AssignedSignals=Temperature
  Bus Selector : BusSelector  OutputSignals=Temperature,Pressure,FluidType,FluidMix,MassFlow
  Heat_Capacity : $bdroot/Basic/Material_Properties/Heat_Capacity  VariantControl=CarlibClassic  INPUTARGUMENTS=state variables (classic)  DEBUGLEVEL=DEBUGLEVEL  MAXTOTALWARNINGS=inf  MAXCONSECUTIVEWARNINGS=inf  WRITETOFILE=0  FILENAME='errors.txt'
  Pipe : $bdroot/Hydraulics/Pipe  dia=0.02  len=10  hgt=5  uloss=100/20/10  cond=0  cwall=1000  t0=20  lin=100/0.2  qua=100/0.2^2  nodes=10
  Product2 : Product  Inputs=**  SaturateOnIntegerOverflow=on  RndMeth=Zero  InputSameDT=on  OutDataTypeStr=Inherit: Same as first input
  Product5 : Product  Inputs=/*  SaturateOnIntegerOverflow=on  RndMeth=Zero  InputSameDT=on  OutDataTypeStr=Inherit: Same as first input
  Sum2 : Sum  InputSameDT=on  OutDataTypeStr=Inherit: Same as first input
  const3 : Constant  Value=20
  isinf : MATLAB Function  TreatAsAtomicUnit=on
  isnan : MATLAB Function  TreatAsAtomicUnit=on
  THB_RC_OUT : Outport
  wires:
  Q_recooling/1 -> Product5/2
  Product2/1 -> Product5/1
  Bus Selector/5 -> Product2/2  "<MassFlow>"
  Heat_Capacity/1 -> Product2/1
  Bus Selector/2 -> Heat_Capacity/2  "<Pressure>"
  Bus Selector/4 -> Heat_Capacity/4  "<FluidMix>"
  Bus Selector/3 -> Heat_Capacity/3  "<FluidType>"
  Bus Selector/1 -> Sum2/1, Heat_Capacity/1  "<Temperature>"
  isnan/1(y) -> isinf/1(u)
  isinf/1(y) -> Sum2/2
  Sum2/1 -> Bus Assignment/2
  Product5/1 -> isnan/1(u)
  Bus Assignment/1 -> Pipe/2
  Pipe/1 -> THB_RC_OUT/1
  const3/1 -> Pipe/1
  THB_RC_IN/1 -> Bus Assignment/1, Bus Selector/1

== system carnot/Source/Chiller/Absorption_Chiller_ddT/Transfer Fcn (with initial states) ==
  In1 : Inport
  State Space : StateSpace  A=A  B=B  C=C  D=Dd  InitialCondition=X0
  Out1 : Outport  InitialOutput=0
  wires:
  In1/1 -> State Space/1
  State Space/1 -> Out1/1

== system carnot/Source/Chiller/Absorption_Chiller_ddT/absorber // condenser ==
  note: Qdot_E + Qdot_G = Qdot_A + Qdot_C
  THBcooler_in : Inport
  Qdot_E_act [W] : Inport  Port=2
  Qdot_G [W] : Inport  Port=3
  on : Inport  Port=4
  Add1 : Sum
  Bus Assignment : BusAssignment  AssignedSignals=Temperature
  Bus Selector : BusSelector  OutputSignals=Temperature,MassFlow,Pressure,FluidType,FluidMix
  Tcooler_out : Subsystem
  prod : Product
  THBcooler : Outport
  t_AC : Outport  Port=2
  wires:
  Tcooler_out/1(Tcooler_out) -> Bus Assignment/2
  Bus Assignment/1 -> THBcooler/1
  prod/1 -> Tcooler_out/3(Qdot_E + Qdot_G)
  Add1/1 -> prod/2
  on/1 -> prod/1
  Qdot_G [W]/1 -> Add1/2
  Qdot_E_act [W]/1 -> Add1/1
  THBcooler_in/1 -> Bus Assignment/1, Bus Selector/1
  Bus Selector/5 -> Tcooler_out/6(mix)  "<FluidMix>"
  Bus Selector/4 -> Tcooler_out/5(fluid)  "<FluidType>"
  Bus Selector/3 -> Tcooler_out/4(p)  "<Pressure>"
  Bus Selector/1 -> t_AC/1, Tcooler_out/1(T)  "<Temperature>"
  Bus Selector/2 -> Tcooler_out/2(mdot)  "<MassFlow>"
